simulink model "FreePC"  (R2024b)
settings: Solver=FixedStepAuto  StartTime=0.0  StopTime=5  FixedStep=0.01  RelTol=1e-3  EnableMultiTasking=on
undefined symbols (not defined in the file or in its folder): barT, D, HIL
libraries: quarc_library x5
settings Model: SimulationMode=external  Creator=kentaroohki  LastModifiedBy=aki
settings SolverCC: AlgebraicLoopSolver=TrustRegion  PositivePriorityOrder=on
settings DataIOCC: SaveOperatingPoint=on  SaveFormat=Structure  SaveOutput=off  SignalLogging=off  DSMLogging=off  InspectSignalLogs=on  SaveTime=off  ReturnWorkspaceOutputs=off
settings DebuggingCC: UnconnectedInputMsg=warning  UnconnectedOutputMsg=warning  UnconnectedLineMsg=warning  ArithmeticOperatorsInVariantConditions=warning
settings ModelReferenceCC: EnableRefExpFcnMdlSchedulingChecks=on
settings SFSimCC: SimUseLocalCustomCode=off  CustomCodeUndefinedFunction=UseInterfaceOnly
settings RTWCC: Description=QUARC Win64 Target Using Toolchain  SystemTargetFile=quarc_win64.tlc  TemplateMakefile=quarc_default_tmf  RTWUseLocalCustomCode=off  Toolchain=QUARC win64 | nmake (64-bit Windows)  BuildConfiguration=Faster Runs  GPUComputeCapability=3.5
settings STFCustomTargetCC: TargetLangStandard=C99 (ISO)  ConcurrentExecutionCompliant=on  GRTInterface=on  UseToolchainInfoCompliant=on  SystemTargetFile=quarc_win64.tlc
settings GRTTargetCC: ParMdlRefBuildCompliant=off  CompOptLevelCompliant=off  CombineOutputUpdateFcns=off  MatFileLogging=off  CPPClassGenCompliant=off  GRTInterface=on  ExtMode=on  ExtModeMexFile=quarc_comm

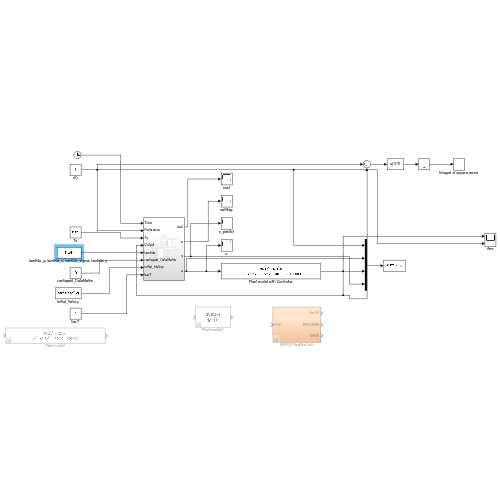
[thumbnail: Simulink's stored preview of the top-level diagram]
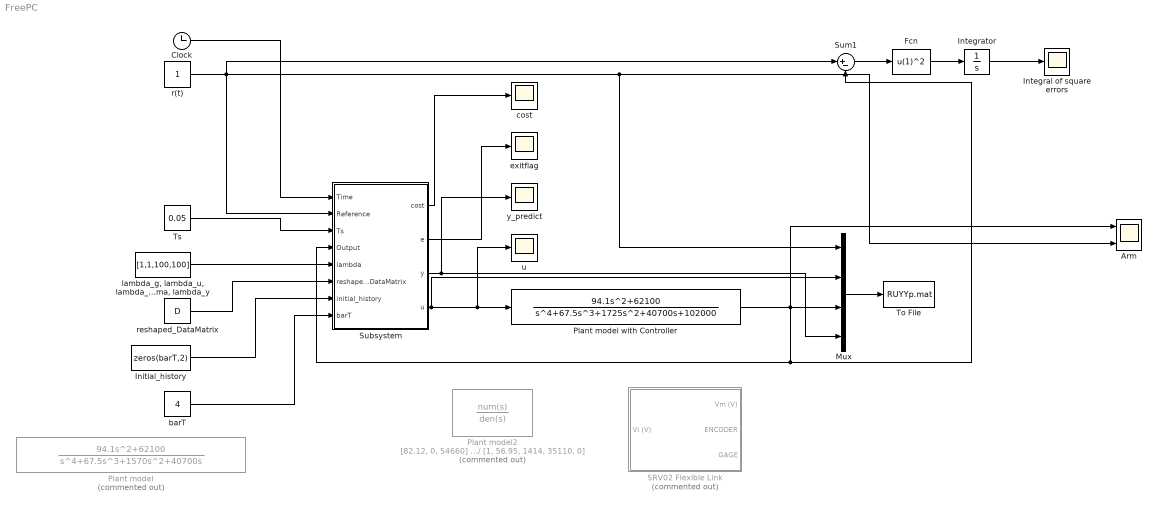
== system FreePC ==
  Arm : Scope  NumInputPorts=2
  Clock : Clock
  Fcn : Fcn  Expr=u(1)^2
  Initial_history : Constant  Value=zeros(barT,2)
  Integral of square errors : Scope
  Integrator : Integrator
  Mux : Mux
  Plant model : TransferFcn  Commented=on  Numerator=[94.1, 0, 62100]  Denominator=[1, 67.5, 1570, 40700, 0]
  Plant model with Controller : TransferFcn  Numerator=[94.1, 0, 62100]  Denominator=[1, 67.5, 1725, 40700, 102000]
  Plant model2 : TransferFcn  Commented=on  Numerator=[82.12, 0, 54660]  Denominator=[1, 56.95, 1414, 35110, 0]
  SRV02 Flexible Link : Subsystem  Commented=on
  Subsystem : Subsystem
  Sum1 : Sum  Inputs=|+-
  To File : ToFile  Filename=RUYYp.mat  MatrixName=RUYYp
  Ts : Constant  Value=0.05
  barT : Constant  Value=4  OutDataTypeStr=int32
  cost : Scope
  exitflag : Scope
  "lambda_g, lambda_u, lambda_sigma, lambda_y " : Constant  Value=[1,1,100,100]
  r(t) : Constant
  reshaped_DataMatrix : Constant  Value=D  VectorParams1D=off
  u : Scope
  y_predict : Scope
  wires:
  Integrator/1 -> Integral of square errors/1
  Mux/1 -> To File/1
  Subsystem/3(y) -> y_predict/1, Mux/4
  barT/1 -> Subsystem/8(barT)
  Initial_history/1 -> Subsystem/7(initial_history)
  Subsystem/2(e) -> exitflag/1
  Fcn/1 -> Integrator/1
  Sum1/1 -> Fcn/1
  reshaped_DataMatrix/1 -> Subsystem/6(reshaped_DataMatrix)
  Clock/1 -> Subsystem/1(Time)
  Ts/1 -> Subsystem/3(Ts)
  Subsystem/1(cost) -> cost/1
  r(t)/1 -> Mux/1, Arm/2, Subsystem/2(Reference), Sum1/1
  "lambda_g, lambda_u, lambda_sigma, lambda_y "/1 -> Subsystem/5(lambda)
  Plant model with Controller/1 -> Sum1/2, Subsystem/4(Output), Arm/1, Mux/3
  Subsystem/4(u) -> Plant model with Controller/1, u/1, Mux/2

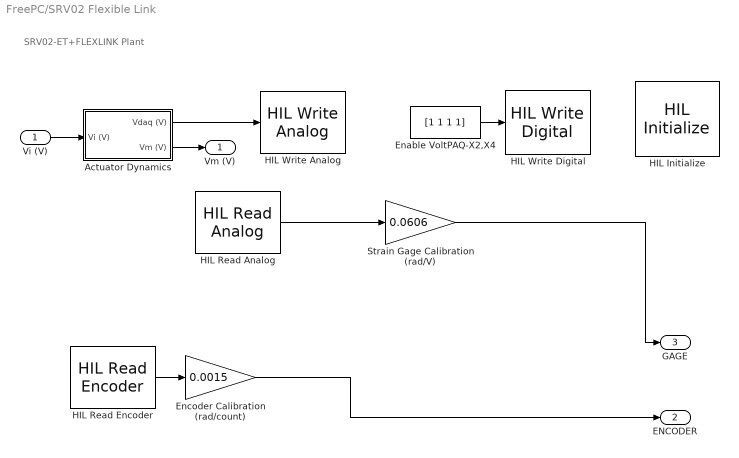
== system FreePC/SRV02 Flexible Link ==
  note: SRV02-ET+FLEXLINK Plant
  Vi (V) : Inport
  Actuator Dynamics : Subsystem
  Enable VoltPAQ-X2,X4 : Constant  Value=[1 1 1 1]
  Encoder Calibration (rad/count) : Gain  Gain=0.0015  SaturateOnIntegerOverflow=on  OutDataTypeStr=Inherit: Same as input  ParamDataTypeStr=Inherit: Same as input
  HIL Initialize : quarc_library/Data Acquisition/Generic/Configuration/HIL Initialize  object_name=HIL-1  board_type=q2_usb  board_number=0  board_options=d0=digital;d1=digital;led=auto;update_rate=normal  exclusive=off  active=off  hardware_clocks=[0:2]  clock_modes=[]  initial_clock_frequencies=[]  set_clock_params_at_start=off  set_clock_params_at_switch_in=off  set_clock_frequencies_at_start=off  set_clock_frequencies_at_switch_in=off  analog_input_channels=[0:1]  analog_input_configurations=[]  analog_input_maximums=10  analog_input_minimums=-10  set_analog_input_params_at_start=on  set_analog_input_params_at_switch_in=off  analog_output_channels=[0:1]  analog_output_maximums=10  analog_output_minimums=-10  initial_analog_outputs=[0]  final_analog_outputs=[0]  watchdog_analog_outputs=0  set_analog_output_params_at_start=on  set_analog_output_params_at_switch_in=off  set_analog_outputs_at_start=on  set_analog_outputs_at_switch_in=off  set_analog_outputs_at_terminate=on  set_analog_outputs_at_switch_out=off  set_analog_outputs_on_watchdog=off  digital_input_channels=[]  digital_output_channels=[0:7]  digital_output_configuration=[]  initial_digital_outputs=[0]  final_digital_outputs=[0]  watchdog_digital_outputs=[0]  set_digital_output_params_at_start=off  set_digital_output_params_at_switch_in=off  set_digital_outputs_at_start=on  set_digital_outputs_at_switch_in=off  set_digital_outputs_at_terminate=on  set_digital_outputs_at_switch_out=off  set_digital_outputs_on_watchdog=off  encoder_channels=[0:1]  quadrature=[4]  encoder_filter_frequency=[]  initial_encoder_counts=[0]  set_encoder_params_at_start=on  set_encoder_params_at_switch_in=off  set_encoder_counts_at_start=on  set_encoder_counts_at_switch_in=off  pwm_channels=[]  pwm_modes=[0]  pwm_frequency=1/0.020  pwm_configuration=[]  pwm_alignment=[]  pwm_polarity=[]  pwm_leading_deadband=[]  pwm_trailing_deadband=[]  initial_pwm_outputs=[0]  final_pwm_outputs=[0]  watchdog_pwm_outputs=[0]  set_pwm_params_at_start=on  set_pwm_params_at_switch_in=off  set_pwm_outputs_at_start=on  set_pwm_outputs_at_switch_in=off  set_pwm_outputs_at_terminate=on  set_pwm_outputs_at_switch_out=off  set_pwm_outputs_on_watchdog=off  other_output_channels=[]  initial_other_outputs=[]  final_other_outputs=[]  watchdog_other_outputs=[]  set_other_outputs_at_start=off  set_other_outputs_at_switch_in=off  set_other_outputs_at_terminate=off  set_other_outputs_at_switch_out=off  set_other_outputs_on_watchdog=off
  HIL Read Analog : quarc_library/Data Acquisition/Generic/Immediate I//O/HIL Read Analog  object_name=HIL-1  channels=0  sample_time=qc_get_step_size  active=on  vector_output=off
  HIL Read Encoder : quarc_library/Data Acquisition/Generic/Immediate I//O/HIL Read Encoder  object_name=HIL-1  channels=0  sample_time=qc_get_step_size  active=on  vector_output=off  data_type_mode=Inherit via back propagation  data_type=double
  HIL Write Analog : quarc_library/Data Acquisition/Generic/Immediate I//O/HIL Write Analog  object_name=HIL-1  channels=0  sample_time=-1  active=off  vector_input=off
  HIL Write Digital : quarc_library/Data Acquisition/Generic/Immediate I//O/HIL Write Digital  object_name=HIL-1  channels=[0:3]  sample_time=-1  active=off  vector_input=on
      settings: SourceProductName=QUARC Targets
  Strain Gage Calibration (rad/V) : Gain  Gain=0.0606  SaturateOnIntegerOverflow=on  OutDataTypeStr=Inherit: Same as input  ParamDataTypeStr=Inherit: Same as input
  Vm (V) : Outport  InitialOutput=0  VectorParamsAs1DForOutWhenUnconnected=off
  ENCODER : Outport  Port=2  InitialOutput=0  VectorParamsAs1DForOutWhenUnconnected=off
  GAGE : Outport  Port=3  InitialOutput=0  VectorParamsAs1DForOutWhenUnconnected=off
  wires:
  Encoder Calibration (rad/count)/1 -> ENCODER/1
  Actuator Dynamics/2(Vm (V)) -> Vm (V)/1
  Actuator Dynamics/1(Vdaq (V)) -> HIL Write Analog/1
  Vi (V)/1 -> Actuator Dynamics/1(Vi (V))
  Enable VoltPAQ-X2,X4/1 -> HIL Write Digital/1
  HIL Read Analog/1 -> Strain Gage Calibration (rad/V)/1
  Strain Gage Calibration (rad/V)/1 -> GAGE/1
  HIL Read Encoder/1 -> Encoder Calibration (rad/count)/1

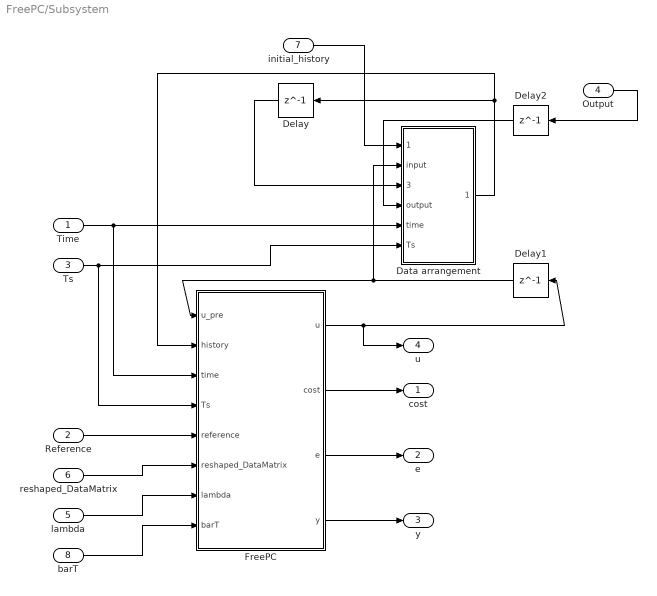
== system FreePC/Subsystem ==
  Time : Inport
  Reference : Inport  Port=2
  Ts : Inport  Port=3
  Output : Inport  Port=4
  lambda : Inport  Port=5
  reshaped_DataMatrix : Inport  Port=6
  initial_history : Inport  Port=7
  barT : Inport  Port=8
  Data arrangement : MATLAB Function  TreatAsAtomicUnit=on
  Delay : Delay  DelayLength=1  InitialCondition=0
  Delay1 : Delay  DelayLength=1  InitialCondition=0
  Delay2 : Delay  DelayLength=1  InitialCondition=0
  FreePC : MATLAB Function  TreatAsAtomicUnit=on
  cost : Outport
  e : Outport  Port=2
  y : Outport  Port=3
  u : Outport  Port=4
  wires:
  Output/1 -> Delay2/1
  Delay1/1 -> FreePC/1(u_pre), Data arrangement/2(input)
  FreePC/4(y) -> y/1
  FreePC/3(e) -> e/1
  barT/1 -> FreePC/8(barT)
  Ts/1 -> FreePC/4(Ts), Data arrangement/6(Ts)
  FreePC/1(u) -> u/1, Delay1/1
  Delay2/1 -> Data arrangement/4(output)
  Data arrangement/1(history) -> FreePC/2(history), Delay/1
  lambda/1 -> FreePC/7(lambda)
  Delay/1 -> Data arrangement/3(history_)
  reshaped_DataMatrix/1 -> FreePC/6(reshaped_DataMatrix)
  initial_history/1 -> Data arrangement/1(initial_history)
  Reference/1 -> FreePC/5(reference)
  FreePC/2(cost) -> cost/1
  Time/1 -> FreePC/3(time), Data arrangement/5(time)

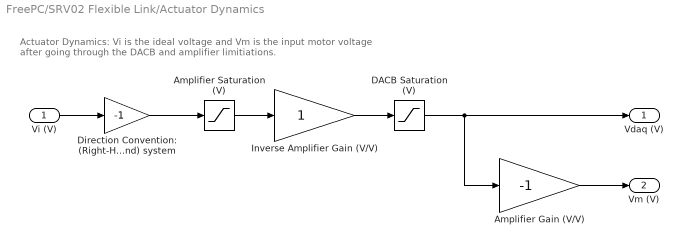
== system FreePC/SRV02 Flexible Link/Actuator Dynamics ==
  note: Actuator Dynamics: Vi is the ideal voltage and Vm is the
      | input motor voltage after going through the DACB and amplifier limitiations.
  Vi (V) : Inport
  Amplifier Saturation (V) : Saturate  UpperLimit=24  LowerLimit=-24
  Amplifier Gain (V/V) : Gain  Gain=-1
  DACB Saturation (V) : Saturate  UpperLimit=10  LowerLimit=-10
  Direction Convention: (Right-Hand) system : Gain  Gain=-1  SaturateOnIntegerOverflow=on  OutDataTypeStr=Inherit: Same as input  ParamDataTypeStr=Inherit: Same as input
  Inverse Amplifier Gain (V/V) : Gain
  Vdaq (V) : Outport  VectorParamsAs1DForOutWhenUnconnected=off
  Vm (V) : Outport  Port=2  VectorParamsAs1DForOutWhenUnconnected=off
  wires:
  Direction Convention: (Right-Hand) system/1 -> Amplifier Saturation (V)/1
  Amplifier Gain (V/V)/1 -> Vm (V)/1
  DACB Saturation (V)/1 -> Vdaq (V)/1, Amplifier Gain (V/V)/1
  Inverse Amplifier Gain (V/V)/1 -> DACB Saturation (V)/1
  Amplifier Saturation (V)/1 -> Inverse Amplifier Gain (V/V)/1
  Vi (V)/1 -> Direction Convention: (Right-Hand) system/1

== matlab function FreePC/Subsystem/FreePC ==
  settings: updateMethod=DISCRETE
  data: u_pre input; history input; time input; Ts input; reference input; reshaped_DataMatrix input; lambda input; u output; cost output; e output; y output; barT input
function [u,cost,e,y]  = fcn(u_pre, history, time, Ts, reference, reshaped_DataMatrix, lambda, barT)

% u_preは最適化によって求まるdouble型の数．制御中はu_preが入力として使われる.
% historyは過去barTステップの「u」と「yの観測値」を記録したもので，history = [u_{k-barT},y_{k-barT}; ... ;u_{k-1},y_{k-1}]
% timeは制御中の現在時刻.
% Tsはステップ幅.
% referenceは定数. y_{0,k}, ..., y_{T-1,k}をreferenceに近づけることがこの制御の目標.
% reshaped_DataMatrixはサイズが2(barT + T) times (2T + 2M + barT) の行列で，データ行列をreshape_DataMatrixで変形したもの.
% barTは参照するuとyの履歴の長さ，Tは予測ホライズンの長さ.
% lambda = [lambda_u, lambda_y, lambda_g, lambda_sigma]は，最適化の目的関数のパラメータ.
% 最適化はここでは二次計画法.


T = size(reshaped_DataMatrix,1)/2 - barT;
M2 = size(reshaped_DataMatrix,2) - 2*T - barT;
referencelist = reference.*ones(T,1);

lambda_g = lambda(1);
lambda_u = lambda(2);
lambda_sigma = lambda(3);
lambda_y = lambda(4);

% 最適化のコスト関数. 文字のおき方はMATLABのquadprogを参照.
H = 2.*blkdiag(lambda_g.*eye(M2),lambda_u.*eye(T),lambda_sigma.*eye(barT),lambda_y.*eye(T));
f = [zeros((T+barT+M2),1); -2*lambda_y.*referencelist];

% 不等式制約（なし）
A = [];
b = [];
    
% xの上限・下限（オプション. x = [g;u;sigma;y]について lb<=x<=ub なる制約を課すことができる. ）
lb = [-100*ones(M2,1); -100*ones(T,1); -1*ones(barT,1); -100*ones(T,1)];
ub = [100*ones(M2,1); 100*ones(T,1); 1*ones(barT,1); 100*ones(T,1)];


if rem(time,Ts) == 0
    
    %等式制約 Aeq x = beq.
    Aeq = reshaped_DataMatrix;
    beq = [history(:,1); zeros(T,1); history(:,2); zeros(T,1)];
    
    % 最適化アルゴリズムを設定
    % 'interior-point-convex' 'trust-region-reflective' 'active-set' の3種類がある.
    options = optimoptions('quadprog', 'Algorithm','active-set','MaxIter',200);
    
    
    % 最適化実行
    [x, fval, exitflag] = quadprog(H, f, A, b, Aeq, beq, lb, ub, 0.1*ones(2*T+M2+barT,1), options);

    u = x(M2+1);
    cost = fval;
    e = exitflag;
    y = x(M2+T+barT+1);

else
    u = u_pre; %次のステップ幅まではu_preを0次ホールドとして入力する．
    y = 0;
    cost = 0;
    e = 0;
end

== matlab function FreePC/Subsystem/Data arrangement ==
  data: initial_history input; input input; history_ input; output input; time input; history output; Ts input
function history = fcn(initial_history, input, history_, output, time, Ts)
% history = [barT past inputs (u), barT past outputs (y)] (barT times 2 matrix)

history = initial_history;

if time > 0
    if rem(time,Ts) == 0
        history = [history_(2:end,:);input,output];
    else
        history = history_;
    end
end
